simulink model "object_frame_impedance"  (R2025a)
settings: Solver=FixedStepDiscrete  StartTime=0.0  StopTime=inf  FixedStep=0.0315/(4*12)  RelTol=1e-3  EnableMultiTasking=on
undefined symbols (not defined in the file or in its folder): f_step, force_step, K_Conn, K_D, K_Or, K_Ot, K_P, ksi, Kx, l_des, Mo, Newton, qd_initial_touch, R_O_Desired, Raphson, sigbuilder_block, t_f_start, torque_step, x_O_desired
libraries: dspmtrx3 x33, dspinverses x1
(part 1 of 6)
settings Model: Creator=konstantinos  LastModifiedBy=kvasios
settings SolverCC: AlgebraicLoopSolver=TrustRegion
settings DataIOCC: LimitDataPoints=on  SaveFormat=Array  SignalLoggingSaveFormat=ModelDataLogs  SaveOutput=off  SaveTime=off  ReturnWorkspaceOutputs=off
settings OptimizationCC: ExpressionDepthLimit=2147483647.0  LifeSpan=inf  SimCompilerOptimization=on
settings DebuggingCC: UnderspecifiedInitializationDetection=Classic  MergeDetectMultiDrivingBlocksExec=none  SolverPrmCheckMsg=warning  FcnCallInpInsideContextMsg=warning  UnconnectedInputMsg=warning  UnconnectedOutputMsg=warning  UnconnectedLineMsg=warning  StateNameClashWarn=warning  SFUnexpectedBacktrackingDiag=warning  SFNoUnconditionalDefaultTransitionDiag=warning  SFExecutionAtInitializationDiag=none  ArithmeticOperatorsInVariantConditions=warning
settings HardwareCC: ProdBitPerPointer=32.0  ProdBitPerSizeT=32.0  ProdBitPerPtrDiffT=32.0  ProdLargestAtomicFloat=None  ProdIntDivRoundTo=Undefined  ProdEndianess=Unspecified  ProdWordSize=32.0  ProdHWDeviceType=32-bit Generic
settings ModelReferenceCC: PropagateSignalLabelsOutOfModel=off
settings SFSimCC: SimUseLocalCustomCode=off  SimParseCustomCode=off  CustomCodeUndefinedFunction=UseInterfaceOnly
settings RTWCC: RTWUseLocalCustomCode=off  GPUComputeCapability=3.5
settings CodeAppCC: StateflowObjectComments=on
settings GRTTargetCC: TargetLangStandard=C89/C90 (ANSI)  CombineOutputUpdateFcns=off  GRTInterface=on
settings ConfigComp: CovMetricSettings=dw  CovSaveCumulativeToWorkspaceVar=on  CovSaveSingleToWorkspaceVar=on  CovExternalEMLEnable=off

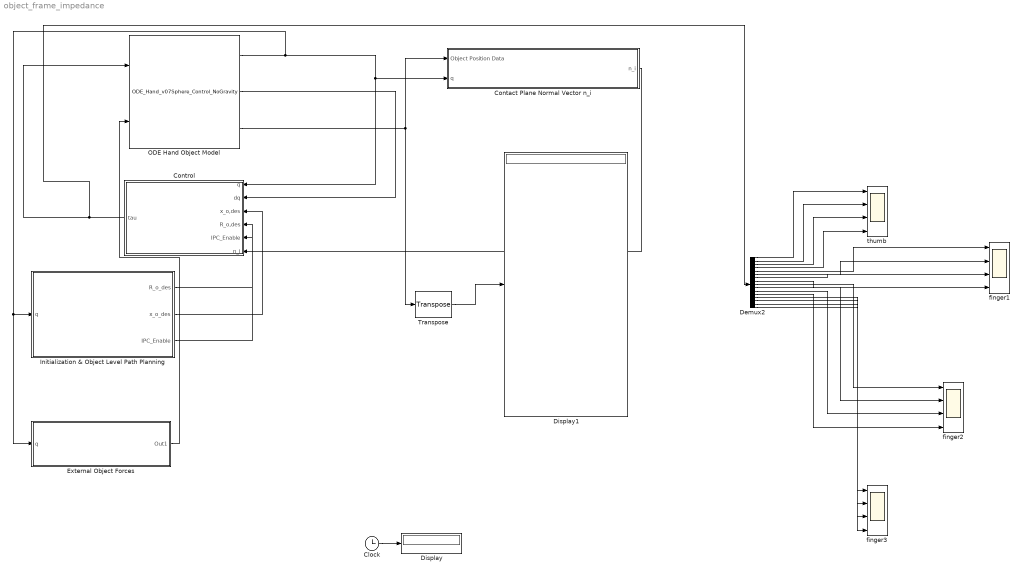
== system object_frame_impedance ==
  Clock : Clock
  Contact Plane Normal Vector n_i : Subsystem
  Control : Subsystem
  Demux2 : Demux  Outputs=16
  Display : Display
  Display1 : Display
  External Object Forces : Subsystem
  Initialization & Object Level Path Planning : Subsystem
  ODE Hand Object Model : S-Function  FunctionName=ODE_Hand_v07Sphere_Control_NoGravity  SFunctionDeploymentMode=off  EnableBusSupport=off
  Transpose : dspmtrx3/Transpose  SystemSampleTime=-1  Hermitian=off  overflowFlag=off
  finger1 : Scope  NumInputPorts=4
      settings: ActiveDisplayYMinimum=-5  ActiveDisplayYMaximum=5  DataLoggingVariableName=tau1_finger
  finger2 : Scope  NumInputPorts=4
      settings: ActiveDisplayYMinimum=-5  ActiveDisplayYMaximum=5  DataLoggingVariableName=tau_finger
  finger3 : Scope  NumInputPorts=4
      settings: ActiveDisplayYMinimum=-5  ActiveDisplayYMaximum=5  DataLoggingVariableName=tau_finger1
  thumb : Scope  NumInputPorts=4
      settings: ActiveDisplayYMinimum=-5  ActiveDisplayYMaximum=5  DataLoggingVariableName=tau_thumb
  wires:
  Clock/1 -> Display/1
  Control/1(tau) -> ODE Hand Object Model/1, Demux2/1
  ODE Hand Object Model/1 -> Control/1(q), Contact Plane Normal Vector n_i/2(q), Initialization & Object Level Path Planning/1(q), External Object Forces/1(q)
  ODE Hand Object Model/2 -> Control/2(dq)
  Initialization & Object Level Path Planning/2(x_o_des) -> Control/3(x_o,des)
  Initialization & Object Level Path Planning/1(R_o_des) -> Control/4(R_o,des)
  Initialization & Object Level Path Planning/3(IPC_Enable) -> Control/5(IPC_Enable)
  Demux2/1 -> thumb/1
  Demux2/2 -> thumb/2
  Demux2/3 -> thumb/3
  Demux2/4 -> thumb/4
  Demux2/5 -> finger1/1
  Demux2/6 -> finger1/2
  Demux2/7 -> finger1/3
  Demux2/8 -> finger1/4
  Demux2/9 -> finger2/1
  Demux2/10 -> finger2/2
  Demux2/11 -> finger2/3
  Demux2/12 -> finger2/4
  Demux2/13 -> finger3/1
  Demux2/14 -> finger3/2
  Demux2/15 -> finger3/3
  Demux2/16 -> finger3/4
  ODE Hand Object Model/3 -> Contact Plane Normal Vector n_i/1(Object Position Data), Transpose/1
  Contact Plane Normal Vector n_i/1(n_i) -> Control/6(n_i)
  Transpose/1 -> Display1/1
  External Object Forces/1(Out1) -> ODE Hand Object Model/2

== system object_frame_impedance/Contact Plane Normal Vector n_i ==
  Object Position Data : Inport
  q : Inport  Port=2
  Cylindrical Object : Subsystem
  Display : Display
  Manual Switch : ManualSwitch
  Sphere : Subsystem
  x_i : MATLABFcn  MATLABFcn=x_i  Output1D=off
  n_i : Outport
  wires:
  Object Position Data/1 -> Sphere/1(In1), Cylindrical Object/1(Position_Orientation)
  Sphere/1(Out1) -> Manual Switch/1
  Cylindrical Object/1(Out1) -> Manual Switch/2
  Manual Switch/1 -> n_i/1
  x_i/1 -> Cylindrical Object/2(x_i), Sphere/2(In2), Display/1
  q/1 -> x_i/1

== system object_frame_impedance/Control ==
  q : Inport
  dq : Inport  Port=2
  x_o,des : Inport  Port=3
  R_o,des : Inport  Port=4
  IPC_Enable : Inport  Port=5
  n_i : Inport  Port=6
  IPC : Subsystem
  Initial_Posture : Subsystem
  MATLAB Fcn : MATLABFcn  MATLABFcn=u  Output1D=off
  Switch : Switch  SaturateOnIntegerOverflow=off  InputSameDT=off
  tau : Outport
  wires:
  dq/1 -> IPC/2(dq), Initial_Posture/2(dq)
  Switch/1 -> tau/1
  x_o,des/1 -> IPC/3(x_o,des)
  R_o,des/1 -> IPC/4(R_o,des)
  IPC/1(tau) -> Switch/1
  IPC_Enable/1 -> Switch/2
  Initial_Posture/1(Out1) -> Switch/3
  q/1 -> MATLAB Fcn/1
  MATLAB Fcn/1 -> IPC/1(q), Initial_Posture/1(q)
  n_i/1 -> IPC/5(n_i)

== system object_frame_impedance/External Object Forces ==
  q : Inport
  Apply Force : Subsystem
  Apply Torque : Subsystem
  Display : Display
  Force--Torque : ManualSwitch  CurrentSetting=0
  Gain : Gain
  Mux1 : Mux
  Mux2 : Mux  Inputs=3
  Mux3 : Mux
  Object Gravity OFF1 : Constant
  Object Gravity ON : Constant  Value=0
  Object_Gravity OFF-ON : ManualSwitch  CurrentSetting=0
  Zero_the Rest : Constant  Value=zeros(1,16-13)
  Out1 : Outport
  wires:
  Object Gravity OFF1/1 -> Object_Gravity OFF-ON/1
  Object Gravity ON/1 -> Object_Gravity OFF-ON/2
  Mux2/1 -> Out1/1, Display/1
  q/1 -> Apply Force/1(In1), Apply Torque/1(In1)
  Zero_the Rest/1 -> Mux2/3
  Object_Gravity OFF-ON/1 -> Mux2/2
  Mux1/1 -> Force--Torque/1
  Mux3/1 -> Force--Torque/2
  Apply Force/1(Out1) -> Mux1/1
  Apply Force/2(Out2) -> Mux1/2
  Apply Force/3(Out3) -> Mux1/3
  Apply Force/4(Out4) -> Mux1/4
  Apply Torque/1(Out1) -> Mux3/1
  Apply Torque/2(Out2) -> Mux3/2
  Apply Torque/3(Out3) -> Mux3/3
  Apply Torque/4(Out4) -> Mux3/4
  Force--Torque/1 -> Gain/1
  Gain/1 -> Mux2/1

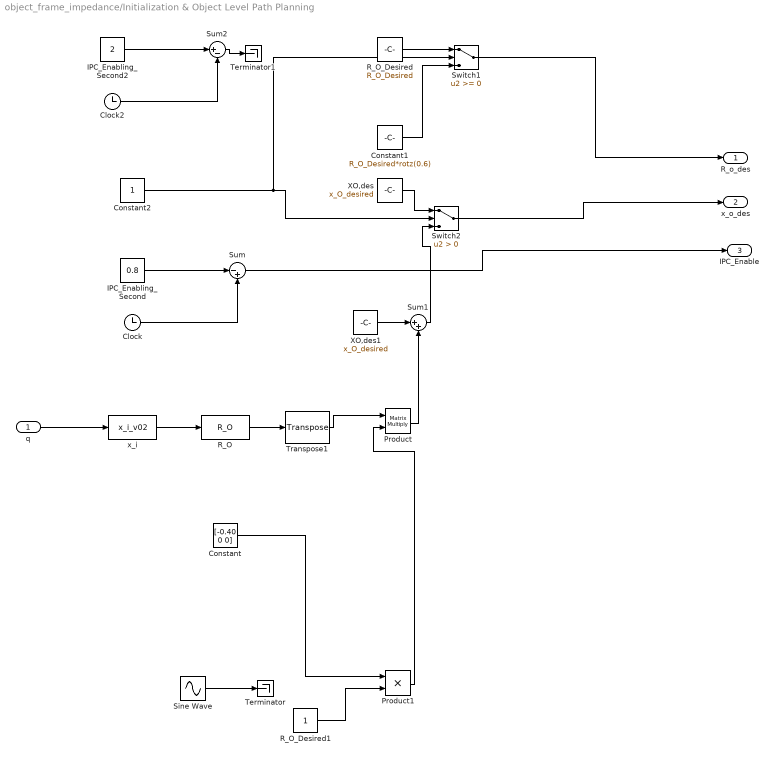
== system object_frame_impedance/Initialization & Object Level Path Planning ==
  q : Inport
  Clock : Clock
  Clock2 : Clock
  Constant : Constant  Value=[-0.40 0 0]
  Constant1 : Constant  Value=R_O_Desired*rotz(0.6)
  Constant2 : Constant
  IPC_Enabling_Second : Constant  Value=0.8
  IPC_Enabling_Second2 : Constant  Value=2
  Product : Product  Multiplication=Matrix(*)  RndMeth=Zero
  Product1 : Product  RndMeth=Zero
  R_O : MATLABFcn  MATLABFcn=R_O  OutputSignalType=real  Output1D=off
  R_O_Desired : Constant  Value=R_O_Desired
  R_O_Desired1 : Constant
  Sine Wave : Sin  Amplitude=0.7  Frequency=4  SampleTime=0
  Sum : Sum  Inputs=|-+
  Sum1 : Sum  Inputs=|++
  Sum2 : Sum  Inputs=|+-
  Switch1 : Switch  SaturateOnIntegerOverflow=off  InputSameDT=off
  Switch2 : Switch  Criteria=u2 > Threshold  SaturateOnIntegerOverflow=off  InputSameDT=off
  Terminator : Terminator
  Terminator1 : Terminator
  Transpose1 : dspmtrx3/Transpose  SystemSampleTime=-1  Hermitian=off  overflowFlag=off
  XO,des : Constant  Value=x_O_desired
  XO,des1 : Constant  Value=x_O_desired
  x_i : MATLABFcn  MATLABFcn=x_i_v02  Output1D=off
  R_o_des : Outport
  x_o_des : Outport  Port=2
  IPC_Enable : Outport  Port=3
  wires:
  Clock/1 -> Sum/2
  IPC_Enabling_Second/1 -> Sum/1
  Sum/1 -> IPC_Enable/1
  R_O_Desired/1 -> Switch1/1
  Switch1/1 -> R_o_des/1
  Switch2/1 -> x_o_des/1
  Constant1/1 -> Switch1/3
  Clock2/1 -> Sum2/2
  IPC_Enabling_Second2/1 -> Sum2/1
  q/1 -> x_i/1
  x_i/1 -> R_O/1
  R_O/1 -> Transpose1/1
  Transpose1/1 -> Product/1
  XO,des1/1 -> Sum1/1
  Product/1 -> Sum1/2
  Sum1/1 -> Switch2/3
  XO,des/1 -> Switch2/1
  Constant/1 -> Product1/1
  Product1/1 -> Product/2
  Sine Wave/1 -> Terminator/1
  R_O_Desired1/1 -> Product1/2
  Constant2/1 -> Switch2/2, Switch1/2
  Sum2/1 -> Terminator1/1

== system object_frame_impedance/Contact Plane Normal Vector n_i/Cylindrical Object ==
  Position_Orientation : Inport
  x_i : Inport  Port=2
  Constant : Constant  Value=zeros(1,12)
  MATLAB Fcn1 : MATLABFcn  MATLABFcn=[u(1,:) u(2,:) u(3,:) u(4,:)]
  Mux : Mux  Inputs=3
  Position : MATLABFcn  MATLABFcn=[u(1:3)]
  Terminator : Terminator
  orientation : MATLABFcn  MATLABFcn=[u(4:6)]
  Out1 : Outport
  wires:
  x_i/1 -> MATLAB Fcn1/1
  Position_Orientation/1 -> Position/1, orientation/1
  Position/1 -> Mux/1
  orientation/1 -> Mux/2
  MATLAB Fcn1/1 -> Mux/3
  Mux/1 -> Terminator/1
  Constant/1 -> Out1/1

== system object_frame_impedance/Contact Plane Normal Vector n_i/Sphere ==
  In1 : Inport
  In2 : Inport  Port=2
  MATLAB Fcn : MATLABFcn  MATLABFcn=Sphere_n_i
  MATLAB Fcn1 : MATLABFcn  MATLABFcn=[u(1,:) u(2,:) u(3,:) u(4,:)]
  MATLAB Fcn2 : MATLABFcn  MATLABFcn=[u(1:3)]
  Mux : Mux  Inputs=2
  Out1 : Outport
  wires:
  MATLAB Fcn/1 -> Out1/1
  In2/1 -> MATLAB Fcn1/1
  MATLAB Fcn1/1 -> Mux/2
  Mux/1 -> MATLAB Fcn/1
  In1/1 -> MATLAB Fcn2/1
  MATLAB Fcn2/1 -> Mux/1

== system object_frame_impedance/Control/IPC ==
  q : Inport
  dq : Inport  Port=2
  x_o,des : Inport  Port=3
  R_o,des : Inport  Port=4
  n_i : Inport  Port=5
  Finger Redundancy Controller : Subsystem
  J : Subsystem
  Object Level Damping(theta) : Subsystem
  "Object Level Stiffnes " : Subsystem
  Sum : Sum  Inputs=|---
  tau : Outport
  wires:
  q/1 -> Object Level Damping(theta)/1(q), J/1(q), "Object Level Stiffnes "/1(q), Finger Redundancy Controller/1(q)
  Sum/1 -> tau/1
  dq/1 -> Object Level Damping(theta)/3(dq), Finger Redundancy Controller/2(dq)
  "Object Level Stiffnes "/1(Out1) -> Sum/2
  Object Level Damping(theta)/1(Out1) -> Sum/3
  J/1(J_Ot) -> "Object Level Stiffnes "/2(J_Ot)
  J/2(J_Or) -> "Object Level Stiffnes "/3(J_Or)
  J/4(J_tot) -> Object Level Damping(theta)/2(J_tot)
  Finger Redundancy Controller/1(tau) -> Sum/1
  x_o,des/1 -> J/2(x_o,des), "Object Level Stiffnes "/5(x_o,des)
  J/3(JConn) -> "Object Level Stiffnes "/4(JConn)
  R_o,des/1 -> "Object Level Stiffnes "/6(R_o,des)
  J/5(JH) -> "Object Level Stiffnes "/7(J_H)
  n_i/1 -> "Object Level Stiffnes "/8(n_i)

== system object_frame_impedance/Control/Initial_Posture ==
  q : Inport
  dq : Inport  Port=2
  Gain : Gain  Gain=K_P
  Gain1 : Gain  Gain=K_D
  Ramp_Singals_qd : Subsystem
  Sum : Sum  Inputs=|--
  Sum1 : Sum  Inputs=|-+
  Out1 : Outport
  wires:
  q/1 -> Sum1/2
  Sum/1 -> Out1/1
  Sum1/1 -> Gain/1
  dq/1 -> Gain1/1
  Gain1/1 -> Sum/1
  Gain/1 -> Sum/2
  Ramp_Singals_qd/1(Out1) -> Sum1/1

== system object_frame_impedance/External Object Forces/Apply Force ==
  In1 : Inport
  Constant : Constant  Value=zeros(1,3)  VectorParams1D=off
  Constant2 : Constant  Value=zeros(1,3)  VectorParams1D=off
  F_x F_y F_z1 : Subsystem
  R_O : MATLABFcn  MATLABFcn=R_O  OutputSignalType=real  Output1D=off
  Transpose : dspmtrx3/Transpose  SystemSampleTime=-1  Hermitian=off  overflowFlag=off
  X_O : MATLABFcn  MATLABFcn=x_O
  x_i : MATLABFcn  MATLABFcn=x_i  Output1D=off
  Out1 : Outport
  Out2 : Outport  Port=2
  Out3 : Outport  Port=3
  Out4 : Outport  Port=4
  wires:
  x_i/1 -> R_O/1, X_O/1
  F_x F_y F_z1/1(Out1) -> Out2/1
  X_O/1 -> Out1/1
  R_O/1 -> Transpose/1
  Transpose/1 -> F_x F_y F_z1/1(xi)
  In1/1 -> x_i/1
  Constant/1 -> Out3/1
  Constant2/1 -> Out4/1

== system object_frame_impedance/External Object Forces/Apply Torque ==
  In1 : Inport
  Subsystem : Subsystem
  Subsystem2 : Subsystem
  Out1 : Outport
  Out2 : Outport  Port=2
  Out3 : Outport  Port=3
  Out4 : Outport  Port=4
  wires:
  Subsystem/1(Out1) -> Out1/1
  Subsystem/2(Out2) -> Out2/1
  Subsystem2/1(Out1) -> Out3/1
  Subsystem2/2(Out2) -> Out4/1
  In1/1 -> Subsystem/1(In1), Subsystem2/1(In1)

== system object_frame_impedance/Control/IPC/Finger Redundancy Controller ==
  q : Inport
  dq : Inport  Port=2
  MATLAB Fcn : MATLABFcn  MATLABFcn=redundancy_controller
  Mux : Mux  Inputs=2
  tau : Outport
  wires:
  dq/1 -> Mux/2
  q/1 -> Mux/1
  Mux/1 -> MATLAB Fcn/1
  MATLAB Fcn/1 -> tau/1

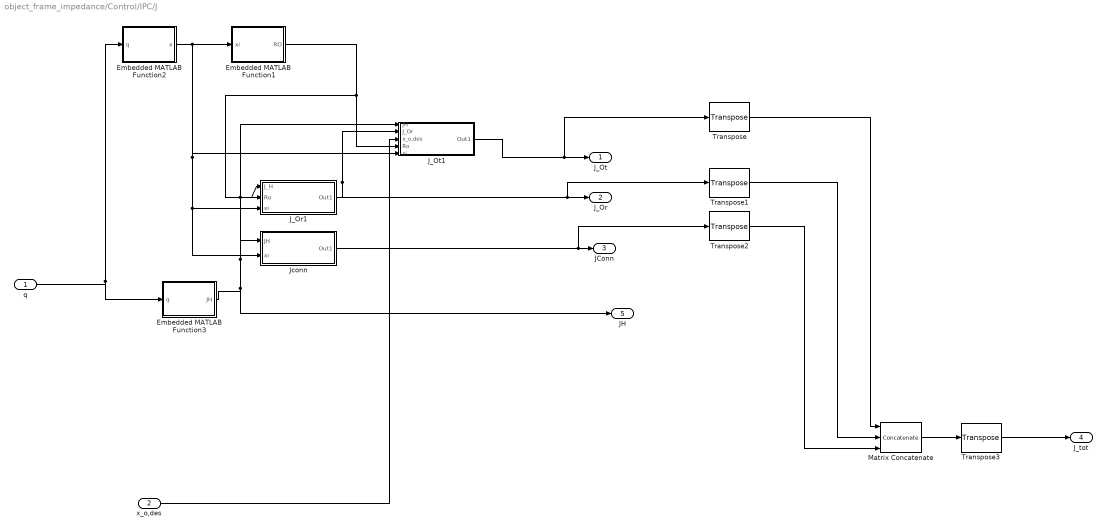
== system object_frame_impedance/Control/IPC/J ==
  q : Inport
  x_o,des : Inport  Port=2
  Embedded MATLAB Function1 : MATLAB Function  TreatAsAtomicUnit=on
  Embedded MATLAB Function2 : MATLAB Function  TreatAsAtomicUnit=on
  Embedded MATLAB Function3 : MATLAB Function  TreatAsAtomicUnit=on
  J_Or1 : Subsystem
  J_Ot1 : Subsystem
  Jconn : Subsystem
  Matrix Concatenate : Concatenate  NumInputs=3  Mode=Multidimensional array  ConcatenateDimension=2
  Transpose{,1..3} (4 alike) : dspmtrx3/Transpose  SystemSampleTime=-1  Hermitian=off  overflowFlag=off
  J_Ot : Outport
  J_Or : Outport  Port=2
  JConn : Outport  Port=3
  J_tot : Outport  Port=4
  JH : Outport  Port=5
  wires:
  Embedded MATLAB Function3/1(JH) -> Jconn/1(JH), J_Or1/1(J_H), J_Ot1/1(JH), JH/1
  J_Or1/1(Out1) -> J_Ot1/2(J_Or), J_Or/1, Transpose1/1
  q/1 -> Embedded MATLAB Function2/1(q), Embedded MATLAB Function3/1(q)
  J_Ot1/1(Out1) -> J_Ot/1, Transpose/1
  Jconn/1(Out1) -> JConn/1, Transpose2/1
  Transpose2/1 -> Matrix Concatenate/3
  Transpose1/1 -> Matrix Concatenate/2
  Transpose/1 -> Matrix Concatenate/1
  Matrix Concatenate/1 -> Transpose3/1
  Transpose3/1 -> J_tot/1
  x_o,des/1 -> J_Ot1/3(x_o,des)
  Embedded MATLAB Function1/1(RO) -> J_Ot1/4(Ro), J_Or1/2(Ro)
  Embedded MATLAB Function2/1(x) -> J_Ot1/5(xi), J_Or1/3(xi), Jconn/2(xi), Embedded MATLAB Function1/1(xi)

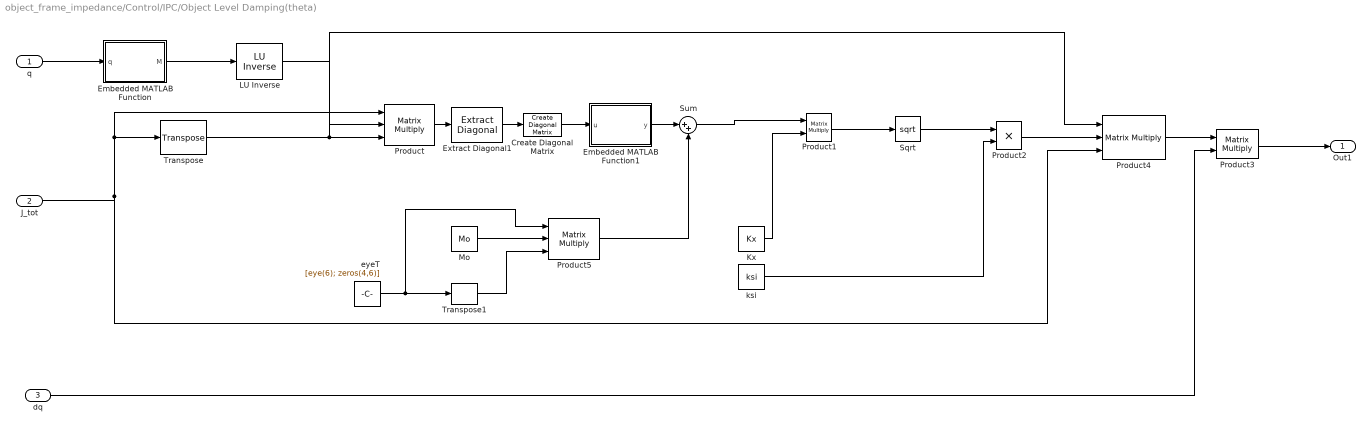
== system object_frame_impedance/Control/IPC/Object Level Damping(theta) ==
  q : Inport
  J_tot : Inport  Port=2
  dq : Inport  Port=3
  " LU Inverse" : dspinverses/ LU Inverse  SystemSampleTime=-1
  Create Diagonal Matrix : dspmtrx3/Create Diagonal Matrix
  Embedded MATLAB Function : MATLAB Function  TreatAsAtomicUnit=on
  Embedded MATLAB Function1 : MATLAB Function  TreatAsAtomicUnit=on
  Extract Diagonal1 : dspmtrx3/Extract Diagonal
  Kx : Constant  Value=Kx
  Mo : Constant  Value=Mo
  Product : Product  Inputs=3  Multiplication=Matrix(*)  RndMeth=Zero
  Product1 : Product  Multiplication=Matrix(*)  RndMeth=Zero
  Product2 : Product  RndMeth=Zero
  Product3 : Product  Multiplication=Matrix(*)  RndMeth=Zero
  Product4 : Product  Inputs=3  Multiplication=Matrix(*)  RndMeth=Zero
  Product5 : Product  Inputs=3  Multiplication=Matrix(*)  RndMeth=Zero
  Sqrt : Sqrt  OutputSignalType=real  AlgorithmType=Newton-Raphson
  Sum : Sum  Inputs=|++
  Transpose : dspmtrx3/Transpose  SystemSampleTime=-1  Hermitian=off  overflowFlag=off
  Transpose1 : dspmtrx3/Transpose  SystemSampleTime=-1  Hermitian=off  overflowFlag=off
  eyeT : Constant  Value=[eye(6); zeros(4,6)]
  ksi : Constant  Value=ksi
  Out1 : Outport
  wires:
  q/1 -> Embedded MATLAB Function/1(q)
  J_tot/1 -> Transpose/1, Product/1, Product4/3
  Transpose/1 -> Product/3, Product4/1
  Embedded MATLAB Function/1(M) -> " LU Inverse"/1
  " LU Inverse"/1 -> Product/2
  Sqrt/1 -> Product2/1
  ksi/1 -> Product2/2
  Product2/1 -> Product4/2
  Product4/1 -> Product3/1
  dq/1 -> Product3/2
  Product3/1 -> Out1/1
  Kx/1 -> Product1/2
  Product1/1 -> Sqrt/1
  eyeT/1 -> Transpose1/1, Product5/1
  Sum/1 -> Product1/1
  Mo/1 -> Product5/2
  Transpose1/1 -> Product5/3
  Product5/1 -> Sum/2
  Product/1 -> Extract Diagonal1/1
  Extract Diagonal1/1 -> Create Diagonal Matrix/1
  Create Diagonal Matrix/1 -> Embedded MATLAB Function1/1(u)
  Embedded MATLAB Function1/1(y) -> Sum/1

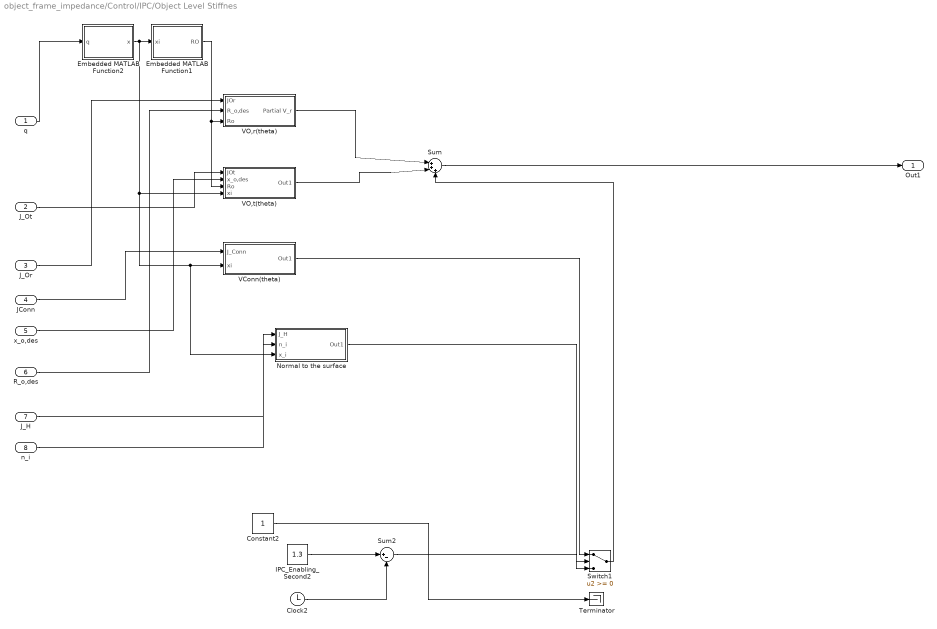
== system object_frame_impedance/Control/IPC/Object Level Stiffnes  ==
  q : Inport
  J_Ot : Inport  Port=2
  J_Or : Inport  Port=3
  JConn : Inport  Port=4
  x_o,des : Inport  Port=5
  R_o,des : Inport  Port=6
  J_H : Inport  Port=7
  n_i : Inport  Port=8
  Clock2 : Clock
  Constant2 : Constant
  Embedded MATLAB Function1 : MATLAB Function  TreatAsAtomicUnit=on
  Embedded MATLAB Function2 : MATLAB Function  TreatAsAtomicUnit=on
  IPC_Enabling_Second2 : Constant  Value=1.3
  Normal to the surface : Subsystem
  Sum : Sum  Inputs=|+++
  Sum2 : Sum  Inputs=|+-
  Switch1 : Switch  SaturateOnIntegerOverflow=off  InputSameDT=off
  Terminator : Terminator
  VConn(theta) : Subsystem
  VO,r(theta) : Subsystem
  VO,t(theta) : Subsystem
  Out1 : Outport
  wires:
  VO,r(theta)/1(Partial V_r) -> Sum/1
  Sum/1 -> Out1/1
  VO,t(theta)/1(Out1) -> Sum/2
  JConn/1 -> VConn(theta)/1(J_Conn)
  J_Ot/1 -> VO,t(theta)/1(JOt)
  J_Or/1 -> VO,r(theta)/1(JOr)
  x_o,des/1 -> VO,t(theta)/2(x_o,des)
  R_o,des/1 -> VO,r(theta)/2(R_o,des)
  Embedded MATLAB Function2/1(x) -> Embedded MATLAB Function1/1(xi), VO,t(theta)/4(xi), VConn(theta)/2(xi), Normal to the surface/3(x_i)
  q/1 -> Embedded MATLAB Function2/1(q)
  Embedded MATLAB Function1/1(RO) -> VO,r(theta)/3(Ro), VO,t(theta)/3(Ro)
  J_H/1 -> Normal to the surface/1(J_H)
  n_i/1 -> Normal to the surface/2(n_i)
  Clock2/1 -> Sum2/2
  IPC_Enabling_Second2/1 -> Sum2/1
  VConn(theta)/1(Out1) -> Switch1/1
  Normal to the surface/1(Out1) -> Switch1/3
  Switch1/1 -> Sum/3
  Constant2/1 -> Terminator/1
  Sum2/1 -> Switch1/2

== system object_frame_impedance/Control/Initial_Posture/Ramp_Singals_qd ==
  Product : Product  RndMeth=Zero
  Ramp : Subsystem  Tag=STV Subsys  LoadFcn=sigbuilder_block('load');  StartFcn=sigbuilder_block('start');  StopFcn=sigbuilder_block('stop');  ClipboardFcn=sigbuilder_block('clipboard');  mask(Sigbuilder block){tuvar=[0:10]}
      mask help: Create and generate interchangeable groups of signals whose waveforms are piecewise linear.
      mask init:
      | if ~strcmp(get_param(bdroot(gcbh),'SimulationStatus'),'stopped') tuvar = sigbuilder_block('maskInit'); end
      settings: CopyFcn=sigbuilder_block('copy');  DeleteFcn=sigbuilder_block('delete');  ModelCloseFcn=sigbuilder_block('modelClose');  PreSaveFcn=sigbuilder_block('preSave');  PauseFcn=sigbuilder_block('pause')  ContinueFcn=sigbuilder_block('continue')  NameChangeFcn=sigbuilder_block('namechange');  OpenFcn=sigbuilder_block('open',[-1260 6 1260 531 ]);  CloseFcn=sigbuilder_block('close');
      mask Display: plot(0, 0, 100, 100,[2, 2, 32, 32, 2], [68, 8, 8, 68, 68],[32, 2], [38, 38], [32, 19, 2],[53, 60, 44], [32, 17, 17, 2],[16, 16, 31, 31]);txt = getActiveGroup(gcbh);text(2, 100, txt,'verticalAlignment', 'top');
  qd_initial_touch : Constant  Value=qd_initial_touch
  Out1 : Outport
  wires:
  Ramp/1(Signal 1) -> Product/1
  qd_initial_touch/1 -> Product/2
  Product/1 -> Out1/1

== system object_frame_impedance/External Object Forces/Apply Force/F_x F_y F_z1 ==
  xi : Inport
  Constant : Constant  Value=0
  Constant1 : Constant  Value=0
  Fx Force Multiplier : Subsystem
  Mux : Mux  Inputs=3
  Product : Product  Multiplication=Matrix(*)  RndMeth=Zero
  Out1 : Outport
  wires:
  Mux/1 -> Product/2
  Product/1 -> Out1/1
  xi/1 -> Product/1
  Fx Force Multiplier/1(Out1) -> Mux/1
  Constant/1 -> Mux/2
  Constant1/1 -> Mux/3

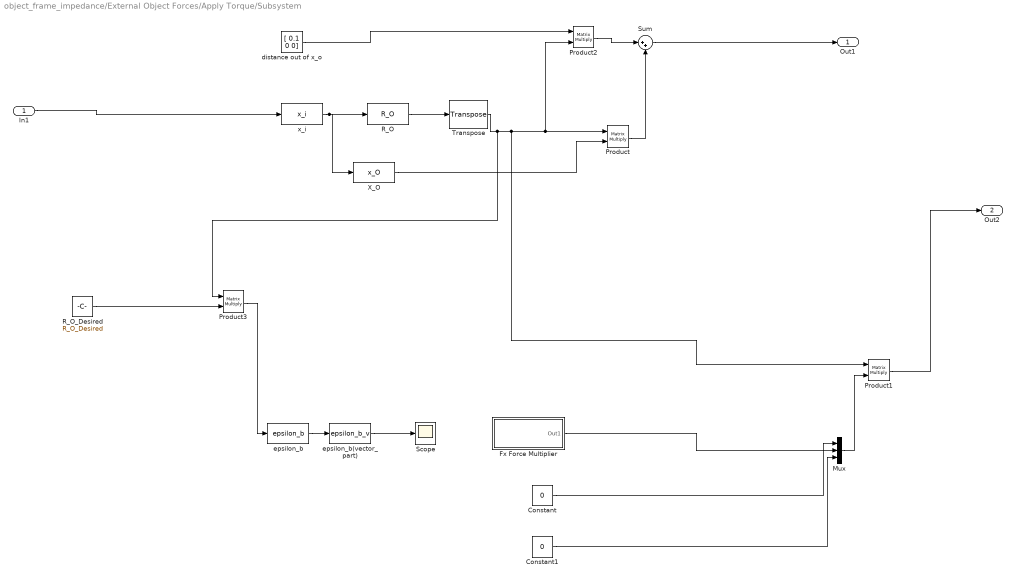
== system object_frame_impedance/External Object Forces/Apply Torque/Subsystem ==
  In1 : Inport
  Constant : Constant  Value=0
  Constant1 : Constant  Value=0
  Fx Force Multiplier : Subsystem
  Mux : Mux  Inputs=3
  Product{,1..3} (4 alike) : Product  Multiplication=Matrix(*)  RndMeth=Zero
  R_O : MATLABFcn  MATLABFcn=R_O  OutputSignalType=real  Output1D=off
  R_O_Desired : Constant  Value=R_O_Desired
  Scope : Scope
      settings: ActiveDisplayYMinimum=-0.325  ActiveDisplayYMaximum=0.05  DataLoggingVariableName=e_b
  Sum : Sum  Inputs=|++
  Transpose : dspmtrx3/Transpose  SystemSampleTime=-1  Hermitian=off  overflowFlag=off
  X_O : MATLABFcn  MATLABFcn=x_O
  distance out of x_o : Constant  Value=[ 0.1 0 0]  VectorParams1D=off
  epsilon_b : MATLABFcn  MATLABFcn=epsilon_b  Output1D=off
  epsilon_b(vector_part) : MATLABFcn  MATLABFcn=epsilon_b_v  Output1D=off
  x_i : MATLABFcn  MATLABFcn=x_i  Output1D=off
  Out1 : Outport
  Out2 : Outport  Port=2
  wires:
  x_i/1 -> R_O/1, X_O/1
  X_O/1 -> Product/2
  R_O/1 -> Transpose/1
  Transpose/1 -> Product1/1, Product/1, Product2/2, Product3/1
  In1/1 -> x_i/1
  Product/1 -> Sum/2
  Mux/1 -> Product1/2
  distance out of x_o/1 -> Product2/1
  Product2/1 -> Sum/1
  Sum/1 -> Out1/1
  Product1/1 -> Out2/1
  Product3/1 -> epsilon_b/1
  epsilon_b/1 -> epsilon_b(vector_part)/1
  epsilon_b(vector_part)/1 -> Scope/1
  R_O_Desired/1 -> Product3/2
  Fx Force Multiplier/1(Out1) -> Mux/2
  Constant/1 -> Mux/1
  Constant1/1 -> Mux/3

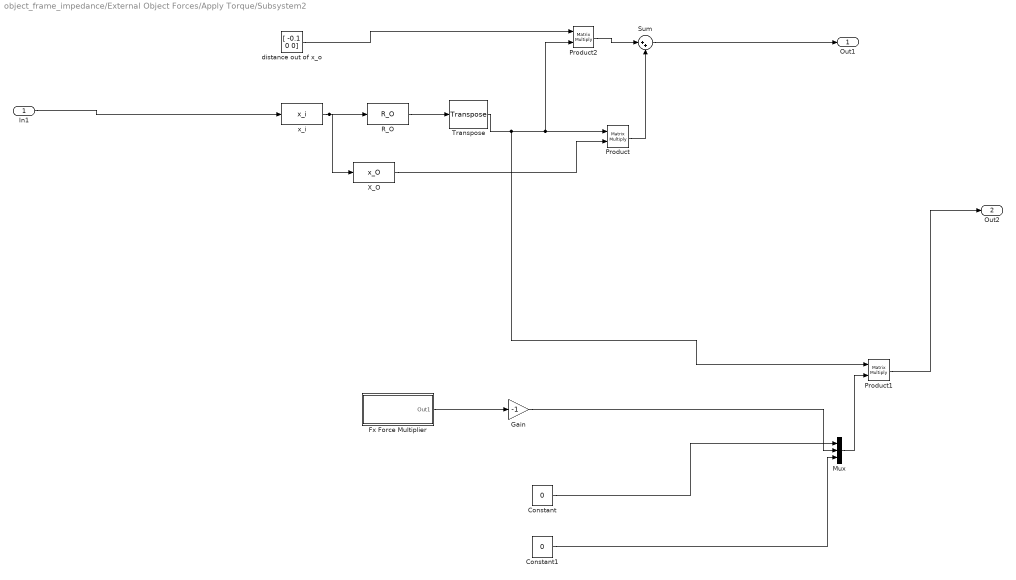
== system object_frame_impedance/External Object Forces/Apply Torque/Subsystem2 ==
  In1 : Inport
  Constant : Constant  Value=0
  Constant1 : Constant  Value=0
  Fx Force Multiplier : Subsystem
  Gain : Gain  Gain=-1
  Mux : Mux  Inputs=3
  Product : Product  Multiplication=Matrix(*)  RndMeth=Zero
  Product1 : Product  Multiplication=Matrix(*)  RndMeth=Zero
  Product2 : Product  Multiplication=Matrix(*)  RndMeth=Zero
  R_O : MATLABFcn  MATLABFcn=R_O  OutputSignalType=real  Output1D=off
  Sum : Sum  Inputs=|++
  Transpose : dspmtrx3/Transpose  SystemSampleTime=-1  Hermitian=off  overflowFlag=off
  X_O : MATLABFcn  MATLABFcn=x_O
  distance out of x_o : Constant  Value="[ -0.1 0   0]"  VectorParams1D=off
  x_i : MATLABFcn  MATLABFcn=x_i  Output1D=off
  Out1 : Outport
  Out2 : Outport  Port=2
  wires:
  x_i/1 -> R_O/1, X_O/1
  X_O/1 -> Product/2
  R_O/1 -> Transpose/1
  Transpose/1 -> Product1/1, Product/1, Product2/2
  In1/1 -> x_i/1
  Product/1 -> Sum/2
  Mux/1 -> Product1/2
  distance out of x_o/1 -> Product2/1
  Product2/1 -> Sum/1
  Sum/1 -> Out1/1
  Product1/1 -> Out2/1
  Fx Force Multiplier/1(Out1) -> Gain/1
  Constant/1 -> Mux/1
  Gain/1 -> Mux/2
  Constant1/1 -> Mux/3

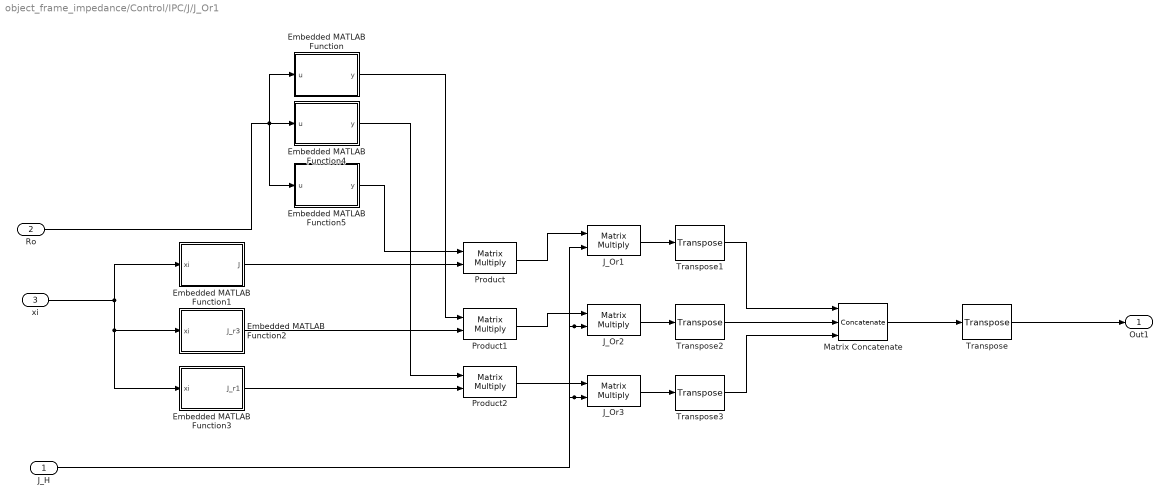
== system object_frame_impedance/Control/IPC/J/J_Or1 ==
  J_H : Inport
  Ro : Inport  Port=2
  xi : Inport  Port=3
  Embedded MATLAB Function : MATLAB Function  TreatAsAtomicUnit=on
  Embedded MATLAB Function1 : MATLAB Function  TreatAsAtomicUnit=on
  Embedded MATLAB Function2 : MATLAB Function  TreatAsAtomicUnit=on
  Embedded MATLAB Function3 : MATLAB Function  TreatAsAtomicUnit=on
  Embedded MATLAB Function4 : MATLAB Function  TreatAsAtomicUnit=on
  Embedded MATLAB Function5 : MATLAB Function  TreatAsAtomicUnit=on
  J_Or1 : Product  Multiplication=Matrix(*)  RndMeth=Zero
  J_Or2 : Product  Multiplication=Matrix(*)  RndMeth=Zero
  J_Or3 : Product  Multiplication=Matrix(*)  RndMeth=Zero
  Matrix Concatenate : Concatenate  NumInputs=3  Mode=Multidimensional array  ConcatenateDimension=2
  Product : Product  Multiplication=Matrix(*)  RndMeth=Zero
  Product1 : Product  Multiplication=Matrix(*)  RndMeth=Zero
  Product2 : Product  Multiplication=Matrix(*)  RndMeth=Zero
  Transpose{,1..3} (4 alike) : dspmtrx3/Transpose  SystemSampleTime=-1  Hermitian=off  overflowFlag=off
  Out1 : Outport
  wires:
  Product/1 -> J_Or1/1
  Product1/1 -> J_Or2/1
  Product2/1 -> J_Or3/1
  J_H/1 -> J_Or2/2, J_Or1/2, J_Or3/2
  Matrix Concatenate/1 -> Transpose/1
  Transpose/1 -> Out1/1
  J_Or1/1 -> Transpose1/1
  J_Or2/1 -> Transpose2/1
  J_Or3/1 -> Transpose3/1
  Transpose2/1 -> Matrix Concatenate/2
  Transpose1/1 -> Matrix Concatenate/1
  Transpose3/1 -> Matrix Concatenate/3
  Embedded MATLAB Function/1(y) -> Product1/1
  Embedded MATLAB Function4/1(y) -> Product2/1
  Embedded MATLAB Function5/1(y) -> Product/1
  Embedded MATLAB Function1/1(J) -> Product/2
  Embedded MATLAB Function2/1(J_r3) -> Product1/2
  Embedded MATLAB Function3/1(J_r1) -> Product2/2
  Ro/1 -> Embedded MATLAB Function/1(u), Embedded MATLAB Function4/1(u), Embedded MATLAB Function5/1(u)
  xi/1 -> Embedded MATLAB Function2/1(xi), Embedded MATLAB Function3/1(xi), Embedded MATLAB Function1/1(xi)

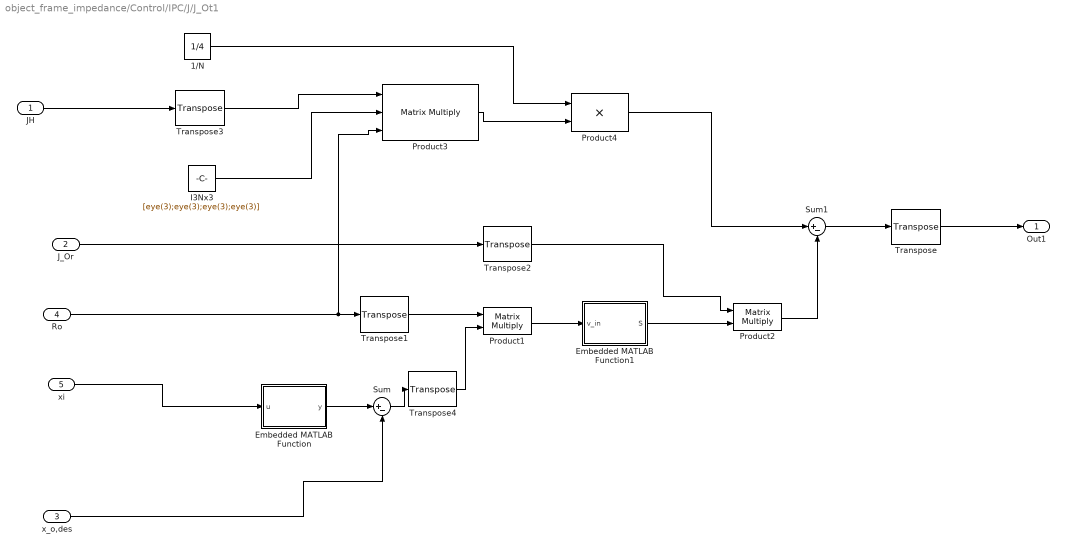
== system object_frame_impedance/Control/IPC/J/J_Ot1 ==
  JH : Inport
  J_Or : Inport  Port=2
  x_o,des : Inport  Port=3
  Ro : Inport  Port=4
  xi : Inport  Port=5
  1/N : Constant  Value=1/4
  Embedded MATLAB Function : MATLAB Function  TreatAsAtomicUnit=on
  Embedded MATLAB Function1 : MATLAB Function  TreatAsAtomicUnit=on
  I3Nx3 : Constant  Value=[eye(3);eye(3);eye(3);eye(3)]
  Product1 : Product  Multiplication=Matrix(*)  RndMeth=Zero
  Product2 : Product  Multiplication=Matrix(*)  RndMeth=Zero
  Product3 : Product  Inputs=3  Multiplication=Matrix(*)  RndMeth=Zero
  Product4 : Product  RndMeth=Zero
  Sum : Sum  Inputs=|+-
  Sum1 : Sum  Inputs=|+-
  Transpose{,1..4} (5 alike) : dspmtrx3/Transpose  SystemSampleTime=-1  Hermitian=off  overflowFlag=off
  Out1 : Outport
  wires:
  Ro/1 -> Transpose1/1, Product3/3
  Embedded MATLAB Function/1(y) -> Sum/1
  x_o,des/1 -> Sum/2
  Transpose1/1 -> Product1/1
  Product1/1 -> Embedded MATLAB Function1/1(v_in)
  Embedded MATLAB Function1/1(S) -> Product2/2
  J_Or/1 -> Transpose2/1
  Transpose2/1 -> Product2/1
  Product2/1 -> Sum1/2
  Sum1/1 -> Transpose/1
  Transpose/1 -> Out1/1
  JH/1 -> Transpose3/1
  Transpose3/1 -> Product3/1
  I3Nx3/1 -> Product3/2
  Product3/1 -> Product4/2
  Product4/1 -> Sum1/1
  1/N/1 -> Product4/1
  xi/1 -> Embedded MATLAB Function/1(u)
  Sum/1 -> Transpose4/1
  Transpose4/1 -> Product1/2

== system object_frame_impedance/Control/IPC/J/Jconn ==
  JH : Inport
  xi : Inport  Port=2
  Embedded MATLAB Function : MATLAB Function  TreatAsAtomicUnit=on
  Product2 : Product  Multiplication=Matrix(*)  RndMeth=Zero
  Transpose : dspmtrx3/Transpose  SystemSampleTime=-1  Hermitian=off  overflowFlag=off
  Transpose1 : dspmtrx3/Transpose  SystemSampleTime=-1  Hermitian=off  overflowFlag=off
  Out1 : Outport
  wires:
  Transpose/1 -> Product2/1
  JH/1 -> Transpose/1
  Product2/1 -> Transpose1/1
  Transpose1/1 -> Out1/1
  xi/1 -> Embedded MATLAB Function/1(xi)
  Embedded MATLAB Function/1(Jc) -> Product2/2

== system object_frame_impedance/Control/IPC/Object Level Stiffnes /Normal to the surface ==
  J_H : Inport
  n_i : Inport  Port=2
  x_i : Inport  Port=3
  F_normal : Constant  Value=F_normal'
  MATLAB Fcn : MATLABFcn  MATLABFcn=[norm(u(1:3)) norm(u(4:6)) norm(u(7:9)) norm(u(10:12))]  Output1D=off
  Null! : MATLABFcn  MATLABFcn=NullSpaceProjection  Output1D=off
  Product : Product  Multiplication=Matrix(*)  RndMeth=Zero
  Product1 : Product  Inputs=3  Multiplication=Matrix(*)  RndMeth=Zero
  Scope1 : Scope
      settings: TimeSpan=10  ActiveDisplayYMinimum=225  ActiveDisplayYMaximum=475  DataLoggingVariableName=f_sn
  Transpose : dspmtrx3/Transpose  SystemSampleTime=-1  Hermitian=off  overflowFlag=off
  gsn : MATLABFcn  MATLABFcn=gsn  Output1D=off
  n : MATLABFcn  MATLABFcn=n  Output1D=off
  r_i : MATLABFcn  MATLABFcn=r_i  Output1D=off
  Out1 : Outport
  wires:
  Product/1 -> Out1/1
  J_H/1 -> Transpose/1
  n_i/1 -> n/1
  r_i/1 -> gsn/1
  Product1/1 -> Product/2, MATLAB Fcn/1
  n/1 -> Product1/2
  F_normal/1 -> Product1/3
  Null!/1 -> Product1/1
  gsn/1 -> Null!/1
  Transpose/1 -> Product/1
  MATLAB Fcn/1 -> Scope1/1
  x_i/1 -> r_i/1

== system object_frame_impedance/Control/IPC/Object Level Stiffnes /VConn(theta) ==
  J_Conn : Inport
  xi : Inport  Port=2
  Embedded MATLAB Function : MATLAB Function  TreatAsAtomicUnit=on
  K_Conn : Constant  Value=K_Conn
  Product : Product  Multiplication=Matrix(*)  RndMeth=Zero
  Product1 : Product  Multiplication=Matrix(*)  RndMeth=Zero
  Sum : Sum  Inputs=|+-
  Transpose : dspmtrx3/Transpose  SystemSampleTime=-1  Hermitian=off  overflowFlag=off
  Transpose1 : dspmtrx3/Transpose  SystemSampleTime=-1  Hermitian=off  overflowFlag=off
  fconn : Scope
      settings: TimeSpan=10  ActiveDisplayYMinimum=150  ActiveDisplayYMaximum=425  DataLoggingVariableName=fConn
  l_des : Constant  Value=l_des
  Out1 : Outport
  wires:
  Embedded MATLAB Function/1(Deltax) -> Sum/1
  l_des/1 -> Sum/2
  Sum/1 -> Product/2
  Product/1 -> Product1/2, fconn/1
  K_Conn/1 -> Product/1
  J_Conn/1 -> Transpose/1
  Transpose/1 -> Product1/1
  Product1/1 -> Transpose1/1
  Transpose1/1 -> Out1/1
  xi/1 -> Embedded MATLAB Function/1(xi)

== system object_frame_impedance/Control/IPC/Object Level Stiffnes /VO,r(theta) ==
  JOr : Inport
  R_o,des : Inport  Port=2
  Ro : Inport  Port=3
  Embedded MATLAB Function2 : MATLAB Function  TreatAsAtomicUnit=on
  K_Or : Constant  Value=K_Or
  Partial V_r(1) : Product  Multiplication=Matrix(*)  RndMeth=Zero
  Product : Product  Multiplication=Matrix(*)  RndMeth=Zero
  Product1 : Product  Multiplication=Matrix(*)  RndMeth=Zero
  Product2 : Product  Multiplication=Matrix(*)  RndMeth=Zero
  Transpose : dspmtrx3/Transpose  SystemSampleTime=-1  Hermitian=off  overflowFlag=off
  Transpose1 : dspmtrx3/Transpose  SystemSampleTime=-1  Hermitian=off  overflowFlag=off
  Transpose2 : dspmtrx3/Transpose  SystemSampleTime=-1  Hermitian=off  overflowFlag=off
  e_b : Scope
      settings: Title=%<mO>  ActiveDisplayYMinimum=-5E-5  ActiveDisplayYMaximum=0.0006  DataLoggingVariableName=e_b
  epsilon_b : MATLABFcn  MATLABFcn=epsilon_b  Output1D=off
  epsilon_b(vector_part) : MATLABFcn  MATLABFcn=epsilon_b_v  Output1D=off
  mO : Scope
      settings: TimeSpan=10  Title=%<mO>  ActiveDisplayYMinimum=-0.3  ActiveDisplayYMaximum=0.2  DataLoggingVariableName=mO
  Partial V_r : Outport
  wires:
  Product1/1 -> Partial V_r(1)/2, mO/1
  K_Or/1 -> Product2/2
  Product2/1 -> Product1/1
  Transpose1/1 -> Partial V_r(1)/1
  Ro/1 -> Transpose/1
  Transpose/1 -> Product/1
  JOr/1 -> Transpose1/1
  Partial V_r(1)/1 -> Transpose2/1
  Transpose2/1 -> Partial V_r/1
  Embedded MATLAB Function2/1(J) -> Product2/1
  R_o,des/1 -> Product/2
  epsilon_b/1 -> epsilon_b(vector_part)/1, Embedded MATLAB Function2/1(e)
  Product/1 -> epsilon_b/1
  epsilon_b(vector_part)/1 -> Product1/2, e_b/1

== system object_frame_impedance/Control/IPC/Object Level Stiffnes /VO,t(theta) ==
  JOt : Inport
  x_o,des : Inport  Port=2
  Ro : Inport  Port=3
  xi : Inport  Port=4
  Embedded MATLAB Function : MATLAB Function  TreatAsAtomicUnit=on
  K_Ot : Constant  Value=K_Ot
  Product{,1..3} (4 alike) : Product  Multiplication=Matrix(*)  RndMeth=Zero
  Scope : Scope
      settings: TimeSpan=7  ActiveDisplayYMinimum=-0.011867678958785381  ActiveDisplayYMaximum=0.02013232104121462  DataLoggingVariableName=x_o
  Sum : Sum  Inputs=|+-
  Transpose : dspmtrx3/Transpose  SystemSampleTime=-1  Hermitian=off  overflowFlag=off
  Transpose1 : dspmtrx3/Transpose  SystemSampleTime=-1  Hermitian=off  overflowFlag=off
  Transpose2 : dspmtrx3/Transpose  SystemSampleTime=-1  Hermitian=off  overflowFlag=off
  fO1 : Scope
      settings: TimeSpan=10  ActiveDisplayYMinimum=-0.25  ActiveDisplayYMaximum=1.75  DataLoggingVariableName=fO
  Out1 : Outport
  wires:
  JOt/1 -> Transpose/1
  Ro/1 -> Transpose1/1
  Embedded MATLAB Function/1(y) -> Sum/1
  Sum/1 -> Product1/2, Product3/2
  Product1/1 -> Product/2
  K_Ot/1 -> Product/1
  Product/1 -> Product2/2, fO1/1
  Transpose/1 -> Product2/1
  Product2/1 -> Transpose2/1
  Transpose2/1 -> Out1/1
  x_o,des/1 -> Sum/2
  Transpose1/1 -> Product1/1, Product3/1
  xi/1 -> Embedded MATLAB Function/1(u)
  Product3/1 -> Scope/1

== system object_frame_impedance/Control/Initial_Posture/Ramp_Singals_qd/Ramp ==
  Demux : Demux  Tag=STV Demux  Outputs=1
      settings: DisplayOption=none
  FromWs : FromWorkspace  Tag=STV FromWs  VariableName=tuvar
  Signal 1 : Outport  Tag=STV Outport
  wires:
  Demux/1 -> Signal 1/1
  FromWs/1 -> Demux/1

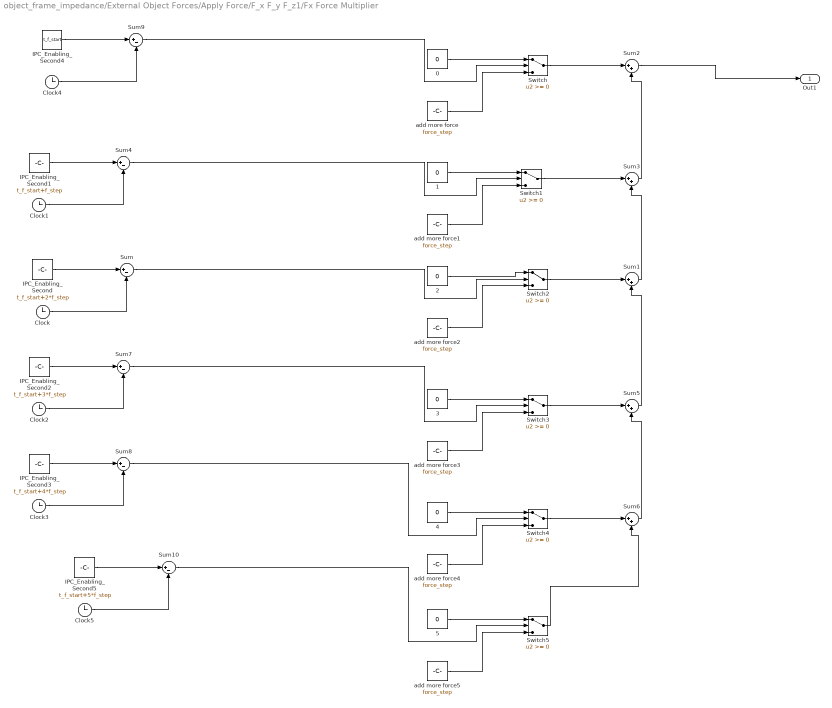
== system object_frame_impedance/External Object Forces/Apply Force/F_x F_y F_z1/Fx Force Multiplier ==
  {0..5} (6 alike) : Constant  Value=0
  Clock{,1..5} (6 alike) : Clock
  IPC_Enabling_Second : Constant  Value=t_f_start+2*f_step
  IPC_Enabling_Second1 : Constant  Value=t_f_start+f_step
  IPC_Enabling_Second2 : Constant  Value=t_f_start+3*f_step
  IPC_Enabling_Second3 : Constant  Value=t_f_start+4*f_step
  IPC_Enabling_Second4 : Constant  Value=t_f_start
  IPC_Enabling_Second5 : Constant  Value=t_f_start+5*f_step
  Sum{,4,7..10} (6 alike) : Sum  Inputs=|+-
  Sum{1..3,5..6} (5 alike) : Sum  Inputs=|++
  Switch{,1..5} (6 alike) : Switch  SaturateOnIntegerOverflow=off  InputSameDT=off
  add more force{,1..5} (6 alike) : Constant  Value=force_step
  Out1 : Outport
  wires:
  0/1 -> Switch/1
  add more force/1 -> Switch/3
  Switch/1 -> Sum2/1
  1/1 -> Switch1/1
  add more force1/1 -> Switch1/3
  Switch1/1 -> Sum3/1
  2/1 -> Switch2/1
  add more force2/1 -> Switch2/3
  Switch2/1 -> Sum1/1
  add more force3/1 -> Switch3/3
  Switch3/1 -> Sum5/1
  4/1 -> Switch4/1
  add more force4/1 -> Switch4/3
  Switch4/1 -> Sum6/1
  5/1 -> Switch5/1
  add more force5/1 -> Switch5/3
  Switch5/1 -> Sum6/2
  Sum3/1 -> Sum2/2
  Sum1/1 -> Sum3/2
  Sum5/1 -> Sum1/2
  Sum6/1 -> Sum5/2
  Clock/1 -> Sum/2
  IPC_Enabling_Second/1 -> Sum/1
  Clock1/1 -> Sum4/2
  IPC_Enabling_Second1/1 -> Sum4/1
  Clock2/1 -> Sum7/2
  IPC_Enabling_Second2/1 -> Sum7/1
  Clock4/1 -> Sum9/2
  IPC_Enabling_Second4/1 -> Sum9/1
  Clock3/1 -> Sum8/2
  IPC_Enabling_Second3/1 -> Sum8/1
  Clock5/1 -> Sum10/2
  IPC_Enabling_Second5/1 -> Sum10/1
  Sum2/1 -> Out1/1
  Sum9/1 -> Switch/2
  Sum4/1 -> Switch1/2
  Sum/1 -> Switch2/2
  3/1 -> Switch3/1
  Sum7/1 -> Switch3/2
  Sum8/1 -> Switch4/2
  Sum10/1 -> Switch5/2

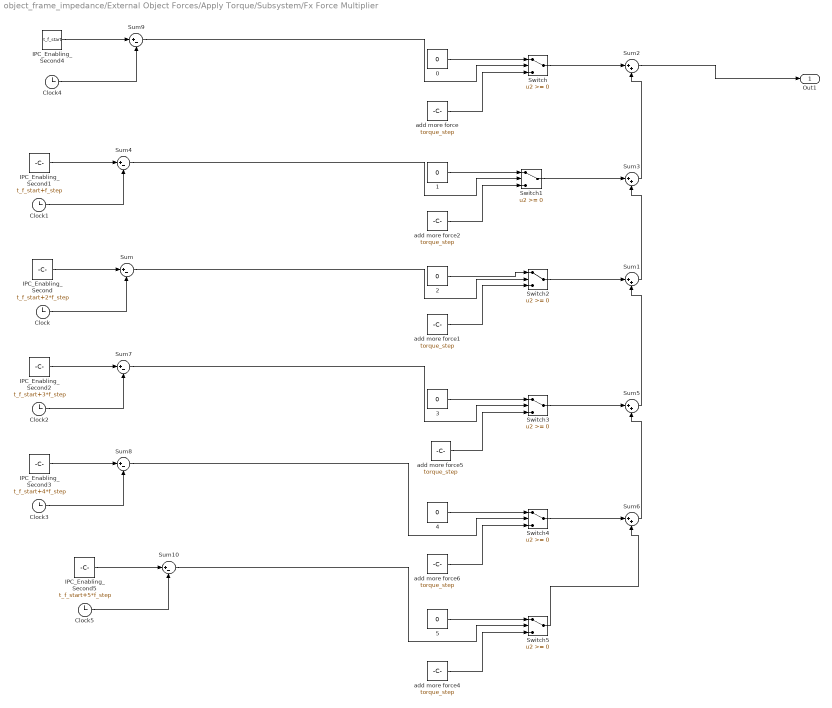
== system object_frame_impedance/External Object Forces/Apply Torque/Subsystem/Fx Force Multiplier ==
  {0..5} (6 alike) : Constant  Value=0
  Clock{,1..5} (6 alike) : Clock
  IPC_Enabling_Second : Constant  Value=t_f_start+2*f_step
  IPC_Enabling_Second1 : Constant  Value=t_f_start+f_step
  IPC_Enabling_Second2 : Constant  Value=t_f_start+3*f_step
  IPC_Enabling_Second3 : Constant  Value=t_f_start+4*f_step
  IPC_Enabling_Second4 : Constant  Value=t_f_start
  IPC_Enabling_Second5 : Constant  Value=t_f_start+5*f_step
  Sum{,4,7..10} (6 alike) : Sum  Inputs=|+-
  Sum{1..3,5..6} (5 alike) : Sum  Inputs=|++
  Switch{,1..5} (6 alike) : Switch  SaturateOnIntegerOverflow=off  InputSameDT=off
  add more force{,1..2,4..6} (6 alike) : Constant  Value=torque_step
  Out1 : Outport
  wires:
  0/1 -> Switch/1
  add more force/1 -> Switch/3
  Switch/1 -> Sum2/1
  1/1 -> Switch1/1
  add more force2/1 -> Switch1/3
  Switch1/1 -> Sum3/1
  2/1 -> Switch2/1
  add more force1/1 -> Switch2/3
  Switch2/1 -> Sum1/1
  add more force5/1 -> Switch3/3
  Switch3/1 -> Sum5/1
  4/1 -> Switch4/1
  add more force6/1 -> Switch4/3
  Switch4/1 -> Sum6/1
  5/1 -> Switch5/1
  add more force4/1 -> Switch5/3
  Switch5/1 -> Sum6/2
  Sum3/1 -> Sum2/2
  Sum1/1 -> Sum3/2
  Sum5/1 -> Sum1/2
  Sum6/1 -> Sum5/2
  Clock/1 -> Sum/2
  IPC_Enabling_Second/1 -> Sum/1
  Clock1/1 -> Sum4/2
  IPC_Enabling_Second1/1 -> Sum4/1
  Clock2/1 -> Sum7/2
  IPC_Enabling_Second2/1 -> Sum7/1
  Clock4/1 -> Sum9/2
  IPC_Enabling_Second4/1 -> Sum9/1
  Clock3/1 -> Sum8/2
  IPC_Enabling_Second3/1 -> Sum8/1
  Clock5/1 -> Sum10/2
  IPC_Enabling_Second5/1 -> Sum10/1
  Sum2/1 -> Out1/1
  Sum9/1 -> Switch/2
  Sum4/1 -> Switch1/2
  Sum/1 -> Switch2/2
  3/1 -> Switch3/1
  Sum7/1 -> Switch3/2
  Sum8/1 -> Switch4/2
  Sum10/1 -> Switch5/2

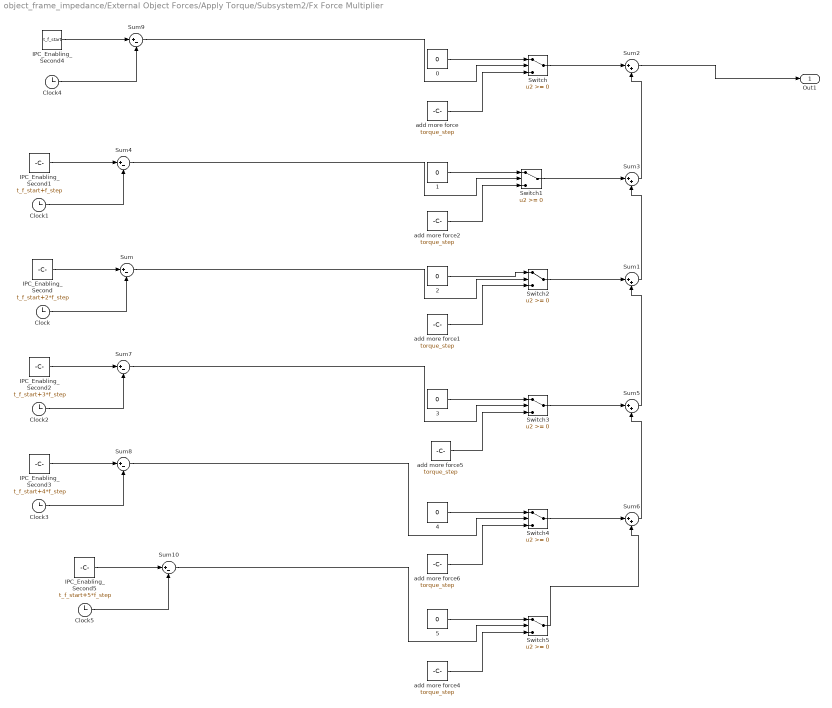
== system object_frame_impedance/External Object Forces/Apply Torque/Subsystem2/Fx Force Multiplier ==
  {0..5} (6 alike) : Constant  Value=0
  Clock{,1..5} (6 alike) : Clock
  IPC_Enabling_Second : Constant  Value=t_f_start+2*f_step
  IPC_Enabling_Second1 : Constant  Value=t_f_start+f_step
  IPC_Enabling_Second2 : Constant  Value=t_f_start+3*f_step
  IPC_Enabling_Second3 : Constant  Value=t_f_start+4*f_step
  IPC_Enabling_Second4 : Constant  Value=t_f_start
  IPC_Enabling_Second5 : Constant  Value=t_f_start+5*f_step
  Sum{,4,7..10} (6 alike) : Sum  Inputs=|+-
  Sum{1..3,5..6} (5 alike) : Sum  Inputs=|++
  Switch{,1..5} (6 alike) : Switch  SaturateOnIntegerOverflow=off  InputSameDT=off
  add more force{,1..2,4..6} (6 alike) : Constant  Value=torque_step
  Out1 : Outport
  wires:
  0/1 -> Switch/1
  add more force/1 -> Switch/3
  Switch/1 -> Sum2/1
  1/1 -> Switch1/1
  add more force2/1 -> Switch1/3
  Switch1/1 -> Sum3/1
  2/1 -> Switch2/1
  add more force1/1 -> Switch2/3
  Switch2/1 -> Sum1/1
  add more force5/1 -> Switch3/3
  Switch3/1 -> Sum5/1
  4/1 -> Switch4/1
  add more force6/1 -> Switch4/3
  Switch4/1 -> Sum6/1
  5/1 -> Switch5/1
  add more force4/1 -> Switch5/3
  Switch5/1 -> Sum6/2
  Sum3/1 -> Sum2/2
  Sum1/1 -> Sum3/2
  Sum5/1 -> Sum1/2
  Sum6/1 -> Sum5/2
  Clock/1 -> Sum/2
  IPC_Enabling_Second/1 -> Sum/1
  Clock1/1 -> Sum4/2
  IPC_Enabling_Second1/1 -> Sum4/1
  Clock2/1 -> Sum7/2
  IPC_Enabling_Second2/1 -> Sum7/1
  Clock4/1 -> Sum9/2
  IPC_Enabling_Second4/1 -> Sum9/1
  Clock3/1 -> Sum8/2
  IPC_Enabling_Second3/1 -> Sum8/1
  Clock5/1 -> Sum10/2
  IPC_Enabling_Second5/1 -> Sum10/1
  Sum2/1 -> Out1/1
  Sum9/1 -> Switch/2
  Sum4/1 -> Switch1/2
  Sum/1 -> Switch2/2
  3/1 -> Switch3/1
  Sum7/1 -> Switch3/2
  Sum8/1 -> Switch4/2
  Sum10/1 -> Switch5/2

== matlab function object_frame_impedance/Control/IPC/J/J_Or1/Embedded MATLAB Function5 ==
  data: u input size=[3 3]; y output
function y = fcn(u)
%#eml

y = u(:,3)';

== matlab function object_frame_impedance/Control/IPC/J/Jconn/Embedded MATLAB Function ==
  data: xi input size=[4 3]; Jc output
%#eml
function Jc=partial_x(xi)

dx =zeros(4,3);
norm_dx=zeros(1,4);


b=(1-(1/4));
a=-1/4;
% a=0;


x1 = xi(1,:);
x2 = xi(2,:);
x3 = xi(3,:);
x4 = xi(4,:);


xO = (1/4)*(x1+x2+x3+x4);
% xO = [0.2000         0    2.09];

% 
dx(1,:)=((x1-xO));
dx(2,:)=((x2-xO));
dx(3,:)=((x3-xO));
dx(4,:)=((x4-xO));

norm_dx(1) = norm(dx(1,:));
norm_dx(2) = norm(dx(2,:));
norm_dx(3) = norm(dx(3,:));
norm_dx(4) = norm(dx(4,:));

partial_delta_x1 = [b*eye(3); a*eye(3); a*eye(3); a*eye(3)];

partial_delta_x2 = [a*eye(3); b*eye(3); a*eye(3); a*eye(3)];

partial_delta_x3 = [a*eye(3); a*eye(3); b*eye(3); a*eye(3)];

partial_delta_x4 = [a*eye(3); a*eye(3); a*eye(3); b*eye(3)];


% size(partial_delta_x1)
% size(dx(1,:))
% size(norm_dx(1))

Jc=[partial_delta_x1*(dx(1,:)'/norm_dx(1)), partial_delta_x2*(dx(2,:)'/norm_dx(2)), ...
    partial_delta_x3*(dx(3,:)'/norm_dx(3)), partial_delta_x4*(dx(4,:)'/norm_dx(4))];

== matlab function object_frame_impedance/Control/IPC/Object Level Stiffnes /VO,r(theta)/Embedded MATLAB Function2 ==
  data: e input; J output
%#eml
function J=Jwe(e)





q0 = e(1); 
q1 = e(2);
q2 = e(3);
q3 = e(4);



% R_O_Desired=[-0.7071    0.7071         0; ...
%     0.7071    0.7071         0; ...
%          0         0   -1.0000];



J = -4*(1/2)*[q0 -q3  q2;...
             q3  q0 -q1;...
            -q2  q1  q0];

== matlab function object_frame_impedance/Control/IPC/Object Level Stiffnes /VConn(theta)/Embedded MATLAB Function ==
  data: xi input size=[4 3]; Deltax output
%#eml
function Deltax=Delta_x(xi)

dx = zeros(1,4);

x1 = xi(1,:);
x2 = xi(2,:);
x3 = xi(3,:);
x4 = xi(4,:);


xO = (1/4)*(x1+x2+x3+x4);
% xO =[0.2000         0    2.0900];


% 
dx(1)=norm((x1-xO));
dx(2)=norm((x2-xO));
dx(3)=norm((x3-xO));
dx(4)=norm((x4-xO));

Deltax=dx';

== matlab function object_frame_impedance/Control/IPC/Object Level Stiffnes /VO,t(theta)/Embedded MATLAB Function ==
  data: u input size=[4 3]; y output
function y = fcn(u)
%#eml

y = ((u(1,:)+u(2,:)+u(3,:)+u(4,:))/4)';

== matlab function object_frame_impedance/Control/IPC/Object Level Stiffnes /Embedded MATLAB Function1 ==
  data: xi input double size=[4 3]; RO output
%#eml
function RO=R_O(xi)



x1 = xi(1,:);
x2 = xi(2,:);
x3 = xi(3,:);
x4 = xi(4,:);

% r1=( xi(1,:)-xi(3,:) )/norm( xi(1,:)-xi(3,:) ) + ...
%     ( xi(2,:)-xi(4,:) )/norm( xi(2,:)-xi(4,:) );

r1=( x1-x3 )/norm( x1-x3 ) + ...
    ( x2-x4 )/norm( x2-x4 );


r1_unit=r1/norm(r1);

% r3= cross( (x1-x3),( x2-x4 ))';

r3= skew( x1-x3 ) * ( x2-x4 )';
r3_unit=r3/norm(r3);

r2_unit = skew(r3_unit)*r1_unit';

l=[r1_unit' r2_unit r3_unit];
RO=l;

== matlab function object_frame_impedance/Control/IPC/J/Embedded MATLAB Function2 ==
  data: q input; x output
%#eml
function x=x_i_v02(q)

x_=zeros(4,3);

rot_base=[0.0000         0   -1.0000;
         0    1.0000         0;
    1.0000         0    0.0000];

L1 = 0.10;
L2 = 1.10;
L3 = 0.60;
L4 = 0.55;

fingers_positions = [-0.70,   0,  L1;...
                      0.60,  0.40,  L1;...
                      0.70,   0,  L1;...
                      0.60,  -0.40, L1];

c=1;
                  
for i=1:4:16,

q1 = q(i);
q2 = q(i+1);
q3 = q(i+2);
q4 = q(i+3);

x_(c,1)=cos(q1) .* (L2 .* cos(q2) + L3 .* cos(q2 + q3) + L4 .*  cos(q2 + q3 + q4));
x_(c,2)=(L2 .* cos(q2) + L3 .* cos(q2 + q3) + L4 .* cos(q2 + q3 + q4)) .* sin(q1);
x_(c,3)= L2 .* sin(q2) + L3 .* sin(q2 + q3) + L4 .* sin(q2 + q3 + q4);

x_(c,:)=rot_base*x_(c,:)'+fingers_positions(c,:)';
c=c+1;
end

x=x_;

== matlab function object_frame_impedance/Control/IPC/Object Level Stiffnes /Embedded MATLAB Function2 ==
  data: q input; x output
%#eml
function x=x_i_v02(q)

x_=zeros(4,3);

rot_base=[0.0000         0   -1.0000;
         0    1.0000         0;
    1.0000         0    0.0000];

L1 = 0.10;
L2 = 1.10;
L3 = 0.60;
L4 = 0.55;

fingers_positions = [-0.70,   0,  L1;...
                      0.60,  0.40,  L1;...
                      0.70,   0,  L1;...
                      0.60,  -0.40, L1];

c=1;
                  
for i=1:4:16,

q1 = q(i);
q2 = q(i+1);
q3 = q(i+2);
q4 = q(i+3);

x_(c,1)=cos(q1) .* (L2 .* cos(q2) + L3 .* cos(q2 + q3) + L4 .*  cos(q2 + q3 + q4));
x_(c,2)=(L2 .* cos(q2) + L3 .* cos(q2 + q3) + L4 .* cos(q2 + q3 + q4)) .* sin(q1);
x_(c,3)= L2 .* sin(q2) + L3 .* sin(q2 + q3) + L4 .* sin(q2 + q3 + q4);

x_(c,:)=rot_base*x_(c,:)'+fingers_positions(c,:)';
c=c+1;
end

x=x_;

== matlab function object_frame_impedance/Control/IPC/J/Embedded MATLAB Function3 ==
  data: q input; JH output
%#eml
function JH=J_H_v02(q)

J=zeros(12,16);

L2 = 1.10;
L3 = 0.60;
L4 = 0.55;

rot_base=[0.0000         0   -1.0000;
         0    1.0000         0;
    1.0000         0    0.0000];

c=1;
for i=1:4:16
q1 = q(i);
q2 = q(i+1);
q3 = q(i+2);
q4 = q(i+3);
    
    
J(c:c+2,i:i+3)=rot_base*[(-1) .* (L2 .* cos(q2) + L3 .* cos(q2 + q3) + L4 .* cos(q2 + q3 + ...
   q4)) .* sin(q1),(-1) .* cos(q1) .* (L2 .* sin(q2) + L3 .* sin(q2  ...
  + q3) + L4 .* sin(q2 + q3 + q4)),(-1) .* cos(q1) .* (L3 .* sin(q2  ...
  + q3) + L4 .* sin(q2 + q3 + q4)),(-1) .* L4 .* cos(q1) .* sin(q2 + ...
   q3 + q4);cos(q1) .* (L2 .* cos(q2) + L3 .* cos(q2 + q3) + L4 .*  ...
  cos(q2 + q3 + q4)),(-1) .* sin(q1) .* (L2 .* sin(q2) + L3 .* sin( ...
  q2 + q3) + L4 .* sin(q2 + q3 + q4)),(-1) .* sin(q1) .* (L3 .* sin( ...
  q2 + q3) + L4 .* sin(q2 + q3 + q4)),(-1) .* L4 .* sin(q1) .* sin( ...
  q2 + q3 + q4);0,cos(q1) .^ 2 .* (L2 .* cos(q2) + L3 .* cos(q2 +  ...
  q3) + L4 .* cos(q2 + q3 + q4)) + (L2 .* cos(q2) + L3 .* cos(q2 +  ...
  q3) + L4 .* cos(q2 + q3 + q4)) .* sin(q1) .^ 2,cos(q1) .* ((-1) .* ...
   L2 .* cos(q1) .* cos(q2) + cos(q1) .* (L2 .* cos(q2) + L3 .* cos( ...
  q2 + q3) + L4 .* cos(q2 + q3 + q4))) + sin(q1) .* ((-1) .* L2 .*  ...
  cos(q2) .* sin(q1) + (L2 .* cos(q2) + L3 .* cos(q2 + q3) + L4 .*  ...
  cos(q2 + q3 + q4)) .* sin(q1)),cos(q1) .* ((-1) .* cos(q1) .* (L2  ...
  .* cos(q2) + L3 .* cos(q2 + q3)) + cos(q1) .* (L2 .* cos(q2) + L3  ...
  .* cos(q2 + q3) + L4 .* cos(q2 + q3 + q4))) + sin(q1) .* ((-1) .*  ...
  (L2 .* cos(q2) + L3 .* cos(q2 + q3)) .* sin(q1) + (L2 .* cos(q2) + ...
   L3 .* cos(q2 + q3) + L4 .* cos(q2 + q3 + q4)) .* sin(q1))];

c=c+3;
end

JH=J;
